simulink model "sim_"  (R2024b)
settings: Solver=VariableStepAuto  StartTime=0.0  StopTime=200  MaxStep=1e-3  RelTol=1e-3
settings Model: Creator=callm  LastModifiedBy=callm
settings DebuggingCC: SignalInfNanChecking=error  SignalRangeChecking=error  AlgebraicLoopMsg=error  CheckMatrixSingularityMsg=error

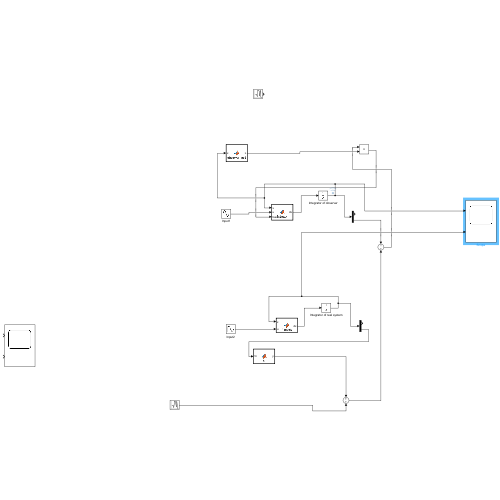
[thumbnail: Simulink's stored preview of the top-level diagram]
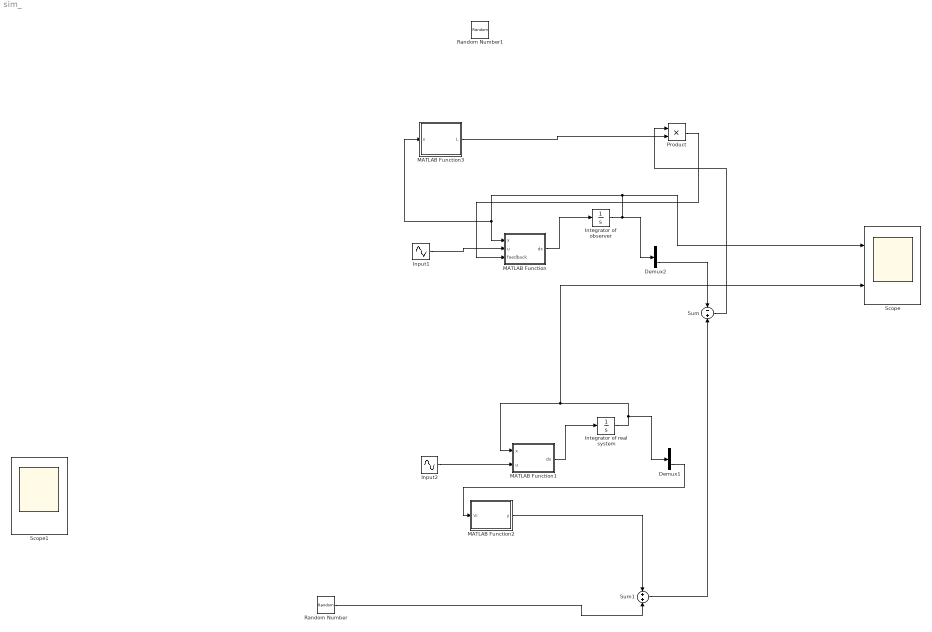
== system sim_ ==
  Demux1 : Demux  Outputs=2
  Demux2 : Demux  Outputs=2
  Input1 : Sin  Bias=100  Frequency=5  SampleTime=0
  Input2 : Sin  Bias=100  Frequency=5  SampleTime=0
  Integrator of observer : Integrator  InitialCondition=[1.9;1.5]  LowerSaturationLimit=[0;0]
  Integrator of real system : Integrator  InitialCondition=[1;100]
  MATLAB Function : MATLAB Function  TreatAsAtomicUnit=on
  MATLAB Function1 : MATLAB Function  TreatAsAtomicUnit=on
  MATLAB Function2 : MATLAB Function  TreatAsAtomicUnit=on
  MATLAB Function3 : MATLAB Function  TreatAsAtomicUnit=on
  Product : Product
  Random Number : RandomNumber  Variance=0.1  Seed=2412  SampleTime=0.1
  Random Number1 : RandomNumber  Variance=0.1  Seed=2412  SampleTime=0.1
  Scope : Scope  NumInputPorts=2
  Scope1 : Scope  NumInputPorts=2
  Sum : Sum  Inputs=-+
  Sum1 : Sum
  wires:
  Input2/1 -> MATLAB Function1/2(u)
  Input1/1 -> MATLAB Function/2(u)
  MATLAB Function/1(dx) -> Integrator of observer/1
  MATLAB Function1/1(dx) -> Integrator of real system/1
  Integrator of real system/1 -> Demux1/1, Scope/2, MATLAB Function1/1(x)
  Demux1/2 -> MATLAB Function2/1(Vi)
  Product/1 -> MATLAB Function/3(feedback)
  Sum/1 -> Product/1
  Integrator of observer/1 -> MATLAB Function3/1(x), MATLAB Function/1(x), Scope/1, Demux2/1
  Demux2/2 -> Sum/1
  Random Number/1 -> Sum1/2
  MATLAB Function3/1(L) -> Product/2
  MATLAB Function2/1(y) -> Sum1/1
  Sum1/1 -> Sum/2

== matlab function sim_/MATLAB Function ==
  data: x input; dx output; u input; feedback input
function dx = f_block(x, u, feedback)
 
%#codegen

% 明确指定维度
assert(isa(x, 'double'));
assert(isa(u, 'double'));
assert(all(size(x) == [2, 1]));


% Duffing 方程参数
Lti=1; Ci=0.05; Ri=96; Pi=0.1;

Iti = x(1);
Vi = x(2);

dx=zeros(2,1);

%Vmin = 80;                 % 你想要的物理最低电压
%Vi_inv = 1 / max(abs(Vi), Vmin);   % 只保护倒数项，不篡改Vi本体

dx(1) = (u - Vi) / Lti;
dx(2) = (Iti ...
        - 0.1 ...
        - (1/Ri)*Vi ...
        - Pi*(1/Vi)) / Ci;


% ---- physical dynamics ----



dx = dx + feedback;    % feedback stays in norm coordinates

end

== matlab function sim_/MATLAB Function3 ==
  data: x input size=[2 1]; L output size=[2 1]
function L  = observer_net(x)
%#codegen

% 明确指定输出维度
L = zeros(2, 1);

Iti = x(1);
Vi = x(2);

persistent F11_grid F12_grid F22_grid
if isempty(F11_grid)
    data = coder.load('P_gridded_interpolants.mat');
    F11_grid = data.F11_grid;
    F12_grid = data.F12_grid;
    F22_grid = data.F22_grid;
end

p11 = F11_grid(Iti, Vi);
p12 = F12_grid(Iti, Vi);
p22 = F22_grid(Iti, Vi);

P = [p11, p12; p12, p22];

L = 1.2*P \ [0; 1];

end

== matlab function sim_/MATLAB Function1 ==
  data: x input; dx output; u input
function dx = f_block(x, u)
%#codegen

% 明确指定维度
assert(isa(x, 'double'));
assert(isa(u, 'double'));
assert(all(size(x) == [2, 1]));

% 明确输出维度

% Duffing 方程参数
Lti=1;
Ci=0.05;
Ri=96;
Pi=0.1;
%Pi=500;

Iti = x(1);
Vi = x(2);
%Vmin = 80;                 % 你想要的物理最低电压
%Vi_inv = 1 / max(abs(Vi), Vmin);   % 只保护倒数项，不篡改Vi本体

dx = zeros(2,1);

dx(1) = (u - Vi) / Lti;
dx(2) = (Iti ...
        - 0.1 ...
        - (1/Ri)*Vi ...
        - Pi*(1/Vi)) / Ci;
                    
end

== matlab function sim_/MATLAB Function2 ==
  data: Vi input; y output size=[1,1]
function y  = h(Vi)

y = Vi;

end
